simulink model "mat2_encoder_mega_V1"  (R2018a)
settings: Solver=FixedStepAuto  StartTime=0.0  StopTime=inf  RelTol=1e-3  EnableMultiTasking=on
libraries: arduinolib x4, simulink x1
settings Model: SimulationMode=external  ExtModeTrigDuration=2  Creator=MU  LastModifiedBy=MU
settings OptimizationCC: EnhancedBackFolding=on  PassReuseOutputArgsThreshold=0  MaxStackSize=64  OptimizeBlockOrder=speed  DifferentSizesBufferReuse=on  OptimizationCustomize=off
settings DebuggingCC: ParameterTunabilityLossMsg=error
settings HardwareCC: ProdBitPerInt=16  ProdBitPerPointer=16  ProdBitPerSizeT=16  ProdBitPerPtrDiffT=16  ProdLargestAtomicFloat=None  ProdWordSize=8  ProdHWDeviceType=Atmel->AVR  UseEmbeddedCoderFeatures=off  UseSimulinkCoderFeatures=off
settings SFSimCC: MATLABDynamicMemAlloc=off
settings RTWCC: SystemTargetFile=ert.tlc  HardwareBoard=Arduino Mega 2560  TLCOptions=-aInlineSetEventsForThisBaseRateFcn=TLC_FALSE -aSuppressMultiTaskScheduler=TLC_FALSE -aRateBasedStepFcn=1  TemplateMakefile=ert_default_tmf  GenerateReport=on  Toolchain=Arduino AVR  BuildConfiguration=Faster Runs  LaunchReport=on
settings CodeAppCC: ForceParamTrailComments=on  OperatorAnnotations=on  MangleLength=10
settings ERTTargetCC: ERTCustomFileBanners=off  SupportContinuousTime=on  SupportNonInlinedSFcns=on  RemoveResetFunc=off  SupportVariableSizeSignals=on  ModelStepFunctionPrototypeControlCompliant=off

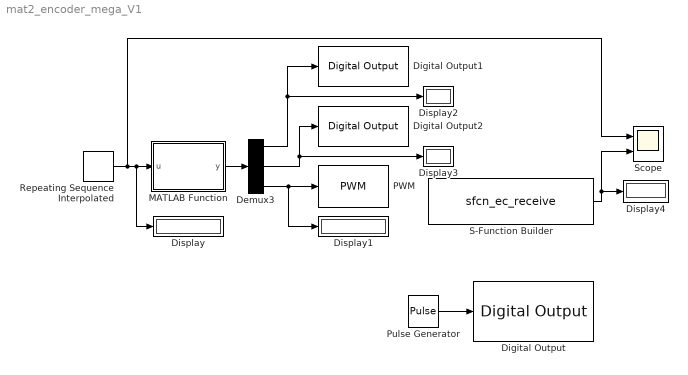
== system mat2_encoder_mega_V1 ==
  Demux3 : Demux  Outputs=3
  Digital Output : arduinolib/Digital Output  pinNumber=13  blockPlatform=arduino
  Digital Output1 : arduinolib/Digital Output  pinNumber=7  blockPlatform=arduino
  Digital Output2 : arduinolib/Digital Output  pinNumber=6  blockPlatform=arduino
  Display{,1..4} (5 alike) : Display
  MATLAB Function : MATLAB Function  TreatAsAtomicUnit=on
  PWM : arduinolib/PWM  pinNumber=5  EnableInputFrequency=off  InitialFrequency=2000  InitialDutyCycle=0  NotificationType=None  blockPlatform=arduino
  Pulse Generator : DiscretePulseGenerator  PulseType=Time based  Period=0.5  PulseWidth=20
  Repeating Sequence Interpolated : simulink/Sources/Repeating Sequence Interpolated  OutValues=[1500 1500 1900 1900 1500 1500 1100 1100 1500 1500].'  TimeValues=[0 1 2 3 4 5 6 7 8 9].'  LookUpMeth=Interpolation-Use End Values  tsamp=0.02  OutMin=[]  OutMax=[]  OutDataTypeStr=double  OutputDataTypeScalingMode=double  OutDataType=fixdt(0,8)  OutScaling=2^-10
  S-Function Builder : S-Function  InitFcn=try, set_param(gcb,'FunctionName','sfcn_ec_receive'), end  FunctionName=sfcn_ec_receive  Parameters=uint8(2),uint8(3)  SFunctionModules=sfcn_ec_receive_wrapper  SFunctionDeploymentMode=off  EnableBusSupport=off  mask(S-Function Builder){}
      mask help: Simulink:masks:SFunctionBuilder_MD
      mask init:
      | val = [[.9  0.75 0.75 1 1 .9 .9 1]',[1 1 0.75 0.75 .9 .9 1 .9]'];try , sys = get_param(gcb,'SfunBuilderFcnName');if isempty(sys), sys = get_param(gcb,'FunctionName'); end,catch, sys = get_param(gcb,'FunctionName'); end
      settings: CopyFcn=set_param(gcbh,'LinkStatus','none')  PreSaveFcn=try, set_param(gcb,'FunctionName','sfcn_ec_receive'), end  OpenFcn=sfunctionwizard(gcbh)
      mask Display: plot(val(:,1),val(:,2)),disp(sys), port_label('output',1,'enc_rpm')
  Scope : Scope  NumInputPorts=2
  wires:
  MATLAB Function/1(y) -> Demux3/1
  Demux3/2 -> Display3/1, Digital Output2/1
  Demux3/3 -> Display1/1, PWM/1
  Demux3/1 -> Display2/1, Digital Output1/1
  Repeating Sequence Interpolated/1 -> Scope/1, Display/1, MATLAB Function/1(u)
  Pulse Generator/1 -> Digital Output/1
  S-Function Builder/1 -> Display4/1, Scope/2

== matlab function mat2_encoder_mega_V1/MATLAB Function ==
  data: u input; y output
function y = fcn(u)
if(u<700) %STOP
        INA1=0;
        INB1=0;
        PWM1=0;
elseif(u<1150) %CW, MAX SPEED
        INA1=1;
        INB1=0;
        PWM1=255;
elseif(u<1450) %CW, Speed control
        INA1=1;
        INB1=0;
        PWM1=(1450-u)/300*255;
elseif(u<1550) %STOP
        INA1=0;
        INB1=0;
        PWM1=0; %Free
        %PWM1=255; %Brake
elseif(u<1850) %CCW, Speed control
        INA1=0;
        INB1=1;
        PWM1=(u-1550)/300*255;
elseif(u<2300) %CCW, MAX SPEED
        INA1=0;
        INB1=1;
        PWM1=255;
else %STOP
        INA1=0;
        INB1=0;
        PWM1=0; 
end
y = [INA1;INB1;PWM1];
